simulink subsystem "SD_Mux"  (R2022b)
settings: Solver=VariableStepAuto  StartTime=0.0  StopTime=10.0  RelTol=1e-3
model mask{a=1, Parameter2=Inherit: Inherit via internal rule}
  mask prompts: a "Amp"; Parameter2 "Data Type"
settings Model: Creator=1111293  LastModifiedBy=qaztr
settings SolverCC: AlgebraicLoopSolver=TrustRegion
settings DebuggingCC: UnconnectedInputMsg=warning  UnconnectedOutputMsg=warning  UnconnectedLineMsg=warning  SFMachineParentedDataDiag=warning
settings ModelReferenceCC: EnableRefExpFcnMdlSchedulingChecks=on
settings RTWCC: DLArmComputeVersion=19.05

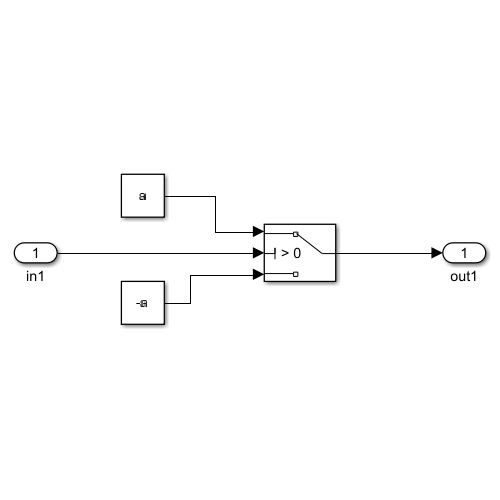
[thumbnail: Simulink's stored preview of the top-level diagram]
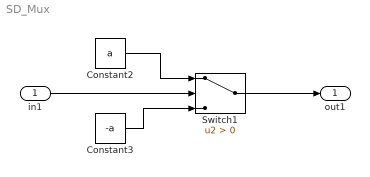
== system SD_Mux ==
  in1 : Inport
  Constant2 : Constant  Value=a
  Constant3 : Constant  Value=-a
  Switch1 : Switch  Criteria=u2 > Threshold  SaturateOnIntegerOverflow=off  InputSameDT=off
  out1 : Outport
  wires:
  Constant2/1 -> Switch1/1
  Switch1/1 -> out1/1
  Constant3/1 -> Switch1/3
  in1/1 -> Switch1/2
